simulink model "IP"  (R2023a)
settings: Solver=VariableStepAuto  StartTime=0.0  StopTime=25  FixedStep=0.1  RelTol=1e-3  AbsTol=1e-3  EnableMultiTasking=on
values from neighbouring files (symbols this model uses):
  A = [0 1 0 0 ... (first row only)    [IP_Parameters.m]
  B = [0;-1/(M*l);0;1/M]    [IP_Parameters.m]
  C = [1 0 1 0 ... (first row only)    [IP_Parameters.m]
  D = [0;0]    [IP_Parameters.m]
  g = 9.81    [IP_Parameters.m]
  kb = 0.031    [IP_Parameters.m]
  Kr = lqr(A,B,Q,R)    [IP_Parameters.m]
  kt = 0.031    [IP_Parameters.m]
  l = 0.36    [IP_Parameters.m]
  M = 2.4    [IP_Parameters.m]
  m = 0.23    [IP_Parameters.m]
  r = 0.006    [IP_Parameters.m]
  reg = lqg(sys,QXU,QWV,QI)    [IP_Parameters.m]
  Rm = 12.5    [IP_Parameters.m]
undefined symbols (not defined in the file or in its folder): b, c, Continuous, Discrete, I, K, KK, sysKF, Time, Vn, X, Y, Z
libraries: sm_lib x36, nesl_utility x20, simulink x14, vrlib x6, ctrlSharedLib x3, slpidlib x1
(part 1 of 2)
settings Model: Creator=M3tal  LastModifiedBy=M3tal
settings SolverCC: AutoScaleAbsTol=off  AlgebraicLoopSolver=TrustRegion  MaxZcPerStep=1
settings DataIOCC: LimitDataPoints=on  MaxDataPoints=10000
settings OptimizationCC: ReuseModelBlockBuffer=off  LifeSpan=inf
settings DebuggingCC: UnconnectedInputMsg=warning  UnconnectedOutputMsg=warning  UnconnectedLineMsg=warning  AllowSymbolicDim=off  SubsystemReferenceDiagnosticForUnitTest=warning  SFUnexpectedBacktrackingDiag=warning  SFNoUnconditionalDefaultTransitionDiag=warning  SFExecutionAtInitializationDiag=none  ArithmeticOperatorsInVariantConditions=warning
settings ModelReferenceCC: EnableRefExpFcnMdlSchedulingChecks=on
settings SFSimCC: SimUseLocalCustomCode=off  CustomCodeUndefinedFunction=UseInterfaceOnly
settings RTWCC: RTWUseLocalCustomCode=off  DLArmComputeVersion=19.05
settings CodeAppCC: StateflowObjectComments=on
settings GRTTargetCC: TargetLangStandard=C89/C90 (ANSI)
settings ConfigComp: CovMetricSettings=dw  CovSaveCumulativeToWorkspaceVar=on  CovSaveSingleToWorkspaceVar=on  CovExternalEMLEnable=off  CovSFcnEnable=off
settings SimscapeCC: SimscapeLogType=all  SimscapeLogSimulationStatistics=on  SimscapeLogDataHistory=10000
settings ExplorerConfigSet: InternalSimMechanicsExplorerSettings="<ExplorerConfiguration><canonicalview>default</canonicalview><AnimationSetting><BasePlaybackSpeed>1.0</BasePlaybackSpeed><PlaybackSpeedFactor>0.25</PlaybackSpeedFactor></AnimationSetting><TilePanel><TileInfo><Tiles Columns=\"1\" Count=\"1\" Rows=\"1\"><Column Weight=\"1\"/><Row Weight=\"1\"/><Tile Height=\"1\" Width=\"1\" X=\"0\" Y=\"0\"/></Tiles></TileInfo><SceneInfo><SceneViewer><BGColor><R>1</R><G>1</G><B>1</B></BGColor><Camera><DoPerspective>off</DoPerspective><Position><X>-0.0931380418765744289</X><Y>-1</Y><Z>0.280046106303800779</Z></Position><Center><X>-0.0931380418765744289</X><Y>-2.77555756156289135e-17</Y><Z>0.280046106303800779</Z></Center><Up><X>0</X><Y>-0</Y><Z>1</Z></Up><ViewLimDist>1</ViewLimDist><YLim>0.450745035862720633</YLim><XLim>0.829412650000000418</XLim></Camera></SceneViewer></SceneInfo></TilePanel><MechEditorPanel><Cameras/><GfxPanelCameraMap/><VideoCreator><PlaybackSpeedRatio>1.0</PlaybackSpeedRatio><FrameRate>30</FrameRate><VideoFormat>Motion JPEG AVI</VideoFormat><FrameSize>auto</FrameSize></VideoCreator></MechEditorPanel></ExplorerConfiguration>"

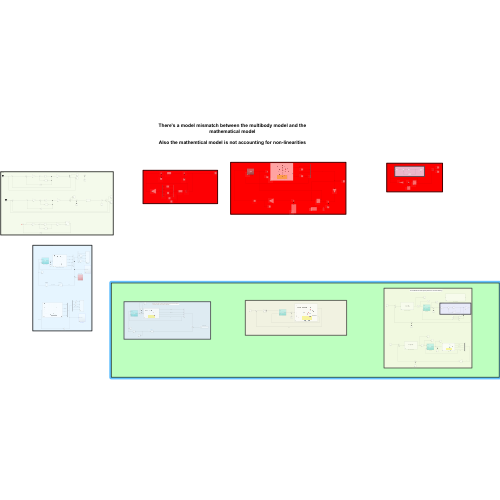
[thumbnail: Simulink's stored preview of the top-level diagram]
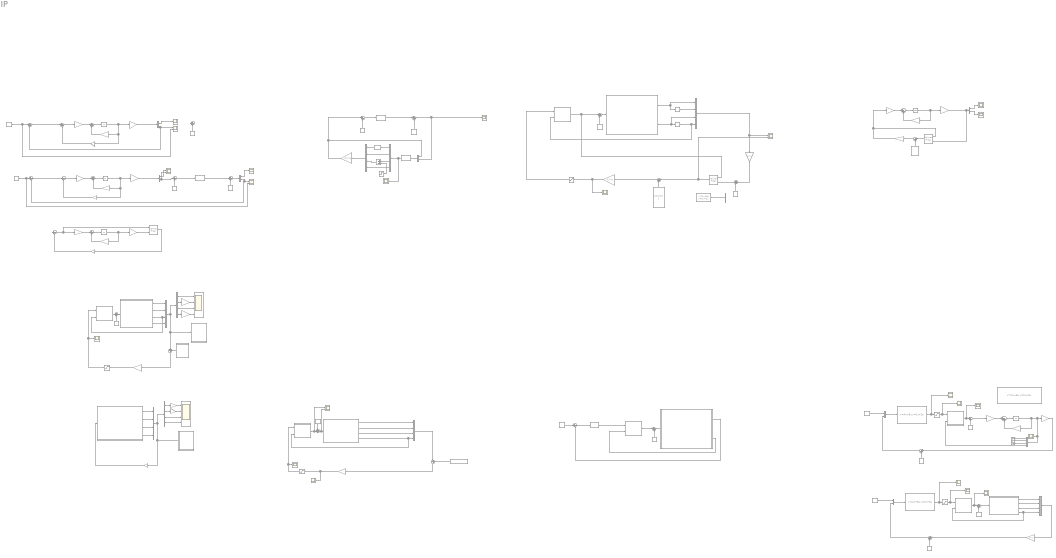
== system IP ==
  note: There's a model mismatch between the multibody model and the mathematical model
      |
      | Also the mathemtical model is not accounting for non-linearities
  note: the model with the state space plant is the one that's working
  note: LQG
  note: Obsolete
  note: nonlinear models in simulink blocks with LQR that i stole
  note: LQG but the G and H matrix are needed
  note: LQG using LQR and KF
  note: LQG Acceptable Results following steve brunton lqg example
  note: PID
  note: When the noise power is incresed the pendulum swerve largely and it loses it's linearzed charecterisitics and the controller doesn't act appropiately
  note: LQR
  note: Plant
  note: Plant
  3D Animation : Subsystem  Commented=on
  3D Animation1 : Subsystem  Commented=on
  Actautor : Subsystem  Commented=on
  Actautor1 : Subsystem  Commented=on
  Actautor2 : Subsystem  Commented=on
  Actautor3 : Subsystem  Commented=on
  Add : Sum  Commented=on  Inputs=+-
  Band-Limited White Noise : simulink/Sources/Band-Limited White Noise  Commented=on  Cov=[1]  Ts=0.1  seed=[23341]
  Band-Limited White Noise{1..2,4,6,11,16..17} (7 alike) : simulink/Sources/Band-Limited White Noise  Commented=on  Cov=[0.1]  Ts=0.1  seed=[23341]
  Band-Limited White Noise{5,8..10} (4 alike) : simulink/Sources/Band-Limited White Noise  Commented=on  Cov=0.1  Ts=0.1  seed=[23341]
  Band-Limited White Noise24 : simulink/Sources/Band-Limited White Noise  Commented=on  Cov=[2]  Ts=0.1  seed=[23341]
  Band-Limited White Noise7 : simulink/Sources/Band-Limited White Noise  Commented=on  Cov=[0.5]  Ts=0.1  seed=[23341]
  Bias1 : Bias  Commented=on  SaturateOnIntegerOverflow=off
  Constant : Constant  Commented=on  Value=[0 0]
  Constant1 : Constant  Commented=on  Value=0
  Constant2 : Constant  Commented=on  Value=[ 0 0 0 0 ]
  Constant3 : Constant  Commented=on  Value=[0 0]
  Demux{,1,3,8} (4 alike) : Demux  Commented=on  Outputs=2
  Demux{4,12..14} (4 alike) : Demux  Commented=on
  Derivative8 : Derivative  Commented=on
  Derivative9 : Derivative  Commented=on
  Desire_state : Subsystem  Commented=on
  Desired state : Constant  Commented=on  Value=[ 0 0 0 0]
  Gain : Gain  Commented=on  Gain=C  Multiplication=Matrix(K*u) (u vector)
  Gain{1,4,9,16,21} (5 alike) : Gain  Commented=on  Gain=A  Multiplication=Matrix(K*u)
  Gain{2,5,10,17,23} (5 alike) : Gain  Commented=on  Gain=C  Multiplication=Matrix(K*u)
  Gain{3,6,11,18,24} (5 alike) : Gain  Commented=on  Gain=B  Multiplication=Matrix(K*u)
  Gain12 : Gain  Commented=on  Gain=K  Multiplication=Matrix(K*u)
  Gain15 : Gain  Commented=on  Gain=Kr  Multiplication=Matrix(K*u) (u vector)
  Gain19 : Gain  Commented=on  Gain=Kr  Multiplication=Matrix(K*u)
  Gain22 : Gain  Commented=on  Gain=-Kr  Multiplication=Matrix(K*u)
  Gain27 : Gain  Commented=on  Gain=Kr  Multiplication=Matrix(K*u) (u vector)
  Gain28 : Gain  Commented=on  Gain=C  Multiplication=Matrix(K*u) (u vector)
  Gain29 : Gain  Commented=on  Gain=KK  Multiplication=Matrix(K*u)
  Gain7 : Gain  Commented=on  Gain=K  Multiplication=Matrix(K*u)
  Gain8 : Gain  Commented=on  Gain=K  Multiplication=Matrix(K*u)
  INPUT : Scope  Commented=on
  IP model using ss : StateSpace  Commented=on  A=A  B=B  C=C  D=D  InitialCondition=0
  Integrator{1..4,6} (5 alike) : Integrator  Commented=on
  Inverted Pendulum System : Subsystem  Commented=on
      mask Display: image('ip_model.png');
  Inverted Pendulum System1 : Subsystem  Commented=on
      mask Display: image('ip_model.png');
  KF using matlab : StateSpace  Commented=on  A=sysKF.A  B=sysKF.B  C=sysKF.C  D=sysKF.D  InitialCondition=0
  KF1 : StateSpace  Commented=on  A=sysKF.A  B=sysKF.B  C=sysKF.C  D=sysKF.D  InitialCondition=0
  Kalman Filter : ctrlSharedLib/Kalman Filter  Commented=on  TimeDomain=Discrete-Time  UseCurrentEstimator=on  ModelSource=LTI State-Space Variable  ModelSourceVariable=ss(0.95,1,1,0,1)  A=0.95  B=1  C=1  D=0  NumberOfStates=1  NumberOfInputs=1  NumberOfOutputs=1  InitialEstimateSource=Dialog  X0=0  P0=10  UseK=off  UseGH=off  NumberOfProcessNoiseInputs=1  G=1  TimeInvariantG=on  H=0  TimeInvariantH=on  Q=0.05  TimeInvariantQ=on  R=1  TimeInvariantR=on  N=0  TimeInvariantN=on  AddInputPort=on  AddEnablePort=off  OutputEstimatedY=off  OutputP=off  Ts=-1
  Kalman Filter1 : ctrlSharedLib/Kalman Filter  Commented=on  TimeDomain=Continuous-Time  UseCurrentEstimator=on  ModelSource=Individual A, B, C, D matrices  ModelSourceVariable=ss(0.95,1,1,0,1)  A=A  B=B  C=C  D=D  NumberOfStates=1  NumberOfInputs=1  NumberOfOutputs=1  InitialEstimateSource=Dialog  X0=0  P0=10  UseK=off  UseGH=off  NumberOfProcessNoiseInputs=1  G=1  TimeInvariantG=on  H=0  TimeInvariantH=on  Q=Vd  TimeInvariantQ=on  R=Vn  TimeInvariantR=on  N=0  TimeInvariantN=on  AddInputPort=on  AddEnablePort=off  OutputEstimatedY=off  OutputP=off  Ts=-1
  Kalman Filter3 : ctrlSharedLib/Kalman Filter  Commented=on  TimeDomain=Continuous-Time  UseCurrentEstimator=on  ModelSource=Individual A, B, C, D matrices  ModelSourceVariable=ss(0.95,1,1,0,1)  A=A  B=B  C=C  D=D  NumberOfStates=1  NumberOfInputs=1  NumberOfOutputs=1  InitialEstimateSource=Dialog  X0=0  P0=10  UseK=off  UseGH=off  NumberOfProcessNoiseInputs=1  G=1  TimeInvariantG=on  H=0  TimeInvariantH=on  Q=0.07  TimeInvariantQ=on  R=1  TimeInvariantR=on  N=0  TimeInvariantN=on  AddInputPort=on  AddEnablePort=off  OutputEstimatedY=off  OutputP=off  Ts=-1
  LQG servo controller : StateSpace  Commented=on  A=reg.A  B=reg.B  C=reg.C  D=reg.D  InitialCondition=0
  LQG servo controller1 : StateSpace  Commented=on  A=reg.A  B=reg.B  C=reg.C  D=reg.D  InitialCondition=0
  LQR_Gain : Gain  Commented=on  Gain=KK  Multiplication=Matrix(K*u)
  Mux{,1,12..13,15,17} (6 alike) : Mux  Commented=on
  Mux{2,5,10..11} (4 alike) : Mux  Commented=on  Inputs=2
  OUTPUT : Scope  Commented=on  NumInputPorts=4
  OUTPUT1 : Scope  Commented=on  NumInputPorts=4
  PID Controller : slpidlib/PID Controller  Commented=on  Controller=PID  Form=Parallel  TimeDomain=Continuous-time  UseExternalTs=off  SampleTime=-1  IntegratorMethod=Forward Euler  FilterMethod=Forward Euler  ControllerParametersSource=internal  P=-3207.65217868692  I=-1870.9153966155  UseKiTs=off  D=-19.0235650193151  N=66.8915557293185  UseFilter=on  TunerSelectOption=Transfer Function Based (PID Tuner App)  InitialConditionSource=internal  InitialConditionForIntegrator=0  InitialConditionForFilter=0  DifferentiatorICPrevScaledInput=0  ExternalReset=none  TrackingMode=off  Kt=1  LimitOutput=on  SatLimitsSource=internal  UpperSaturationLimit=24  LowerSaturationLimit=-24  LinearizeAsGain=on  AntiWindupMode=clamping  Kb=1  LimitIntegrator=off  UpperIntegratorSaturationLimit=24  LowerIntegratorSaturationLimit=-24  POutMin=[]  POutMax=[]  IOutMin=[]  IOutMax=[]  DOutMin=[]  DOutMax=[]  NOutMin=[]  NOutMax=[]  SumOutMin=[]  SumOutMax=[]  SaturationOutMin=[]  SaturationOutMax=[]  PParamMin=[]  PParamMax=[]  IParamMin=[]  IParamMax=[]  DParamMin=[]  DParamMax=[]  NParamMin=[]  NParamMax=[]  KbParamMin=[]  KbParamMax=[]  KtParamMin=[]  KtParamMax=[]  KbOutMin=[]  KbOutMax=[]  KtOutMin=[]  KtOutMax=[]  IntegratorOutMin=[]  IntegratorOutMax=[]  FilterOutMin=[]  FilterOutMax=[]  SumI1OutMin=[]  SumI1OutMax=[]  SumI2OutMin=[]  SumI2OutMax=[]  SumI3OutMin=[]  SumI3OutMax=[]  SumI4OutMin=[]  SumI4OutMax=[]  SumDOutMin=[]  SumDOutMax=[]  DifferentiatorOutMin=[]  DifferentiatorOutMax=[]  FilterDiffOutCoefMin=[]  FilterDiffOutCoefMax=[]  ReciprocalOutMin=[]  ReciprocalOutMax=[]  SumDenOutMin=[]  SumDenOutMax=[]  SumNumOutMin=[]  SumNumOutMax=[]  DivideOutMin=[]  DivideOutMax=[]  UdiffTsProdOutMin=[]  UdiffTsProdOutMax=[]  NTsProdOutMin=[]  NTsProdOutMax=[]  UintegralTsProdOutMin=[]  UintegralTsProdOutMax=[]  UngainTsProdOutMin=[]  UngainTsProdOutMax=[]  ClampingZeroOutDataTypeStr=Inherit: Inherit via back propagation  ClampingZeroOutMin=[]  ClampingZeroOutMax=[]  FilterDenConstantOutDataTypeStr=Inherit: Inherit via back propagation  FilterDenConstantOutMin=[]  FilterDenConstantOutMax=[]  PCopyOutDataTypeStr=Inherit: Inherit via back propagation  PCopyOutMin=[]  PCopyOutMax=[]  NCopyOutDataTypeStr=Inherit: Inherit via back propagation  NCopyOutMin=[]  NCopyOutMax=[]  IntegratorContinuousStateAttributes=''  IntegratorStateMustResolveToSignalObject=off  IntegratorRTWStateStorageClass=Auto  FilterContinuousStateAttributes=''  FilterStateMustResolveToSignalObject=off  FilterRTWStateStorageClass=Auto  ParallelPVariant=InternalParameters  IdealPVariant=Disabled  IVariant=InternalParameters  DVariant=InternalParameters  IntegratorVariant=Continuous  SatVariant=Enabled  AWVariant=ContClampingParallel  PCopyVariant=Disabled  TRVariant=Disabled  FdbkBlocksVariant=Forward  IdealPFdbkVariant=Disabled  SatFdbkVariant=Disabled  DerivativeFilterVariant=ContFilter  NVariant=InternalParameters  NCopyVariant=Disabled  FilterICVariant=InternalICsFilter  IntegratorICVariant=InternalICs  ExternalResetVariant=Disabled  TRSumVariant=Passthrough  SumFdbkVariant=Disabled  SumVariant=Sum_PID  TsampFilterVariant=InternalTs  TsampNgainVariant=Passthrough  TsampIntegralVariant=Disabled_SignalSpec  ExternalSaturationOutDataTypeStr=Inherit: Same as second input
  Plant : Subsystem  Commented=on
      mask Display: image('Annotation 2024-07-04 030345.png'); % Use "Edit Image" on toolstrip to change.
  Plant1 : Subsystem  Commented=on
      mask Display: image('Annotation 2024-07-04 030345.png'); % Use "Edit Image" on toolstrip to change.
  Plant2 : Subsystem  Commented=on
      mask Display: image('Annotation 2024-07-04 030345.png'); % Use "Edit Image" on toolstrip to change.
  Plant9 : Subsystem  Commented=on
      mask Display: image('Annotation 2024-07-04 030345.png'); % Use "Edit Image" on toolstrip to change.
  Plant_in_SSblock : StateSpace  Commented=on  A=A  B=B  C=C  D=D  InitialCondition=0
  R2D : Gain  Commented=on  Gain=180/pi
  R2D1 : Gain  Commented=on  Gain=180/pi
  REf Vs x : Scope  Commented=on  NumInputPorts=2
  Radian_to_Degre : Gain  Commented=on  Gain=180/pi
  Radian_to_Degree : Gain  Commented=on  Gain=180/pi
  Saturation{,1..3} (4 alike) : Saturate  Commented=on  UpperLimit=24  LowerLimit=-24
  Scope{,1,9,18} (4 alike) : Scope  Commented=on  NumInputPorts=2
  Scope{3..8,10..12,14..17,19} (14 alike) : Scope  Commented=on
  Signal Generator : SignalGenerator  Commented=on  WaveForm=square  Units=rad/sec
  Signal Generator1 : SignalGenerator  Commented=on  WaveForm=square  Units=rad/sec
  State-Space : StateSpace  Commented=on  A=A  B=B  C=C  D=D  InitialCondition=0
  Step : Step  Commented=on  Time=10  After=20  SampleTime=0
  Sum{,2..4,8..9,13,15..16,20..22,24..25,33..34,43,46} (18 alike) : Sum  Commented=on  Inputs=|++
  Sum{1,5..7,11..12} (6 alike) : Sum  Commented=on  Inputs=|+-
  Sum{14,17,19,45} (4 alike) : Sum  Commented=on  Inputs=|-+
  Sum18 : Sum  Commented=on  Inputs=++|
  Terminator : Terminator  Commented=on
  Terminator1 : Terminator  Commented=on
  Terminator2 : Terminator  Commented=on
  Volatge_to_Force : Subsystem  Commented=on
  Volatge_to_Force1 : Subsystem  Commented=on
  Voltage Saturation : Saturate  Commented=on  UpperLimit=24  LowerLimit=-24
  Zero : Constant  Commented=on  Value=[ 0 0 0 0]  OutDataTypeStr=Inherit: Inherit via back propagation
  theta : Scope  Commented=on
  theta2 : Scope  Commented=on
  wires:
  Sum1/1 -> PID Controller/1
  Constant1/1 -> Sum1/1
  Signal Generator/1 -> Sum5/1, REf Vs x/2
  State-Space/1 -> Sum4/1
  Band-Limited White Noise1/1 -> Sum4/2
  Sum4/1 -> Demux/1
  Demux/1 -> theta/1
  Demux/2 -> Sum5/2, REf Vs x/1
  ? -> Sum6/1
  Gain6/1 -> Sum3/1
  Gain4/1 -> Sum3/2
  Integrator1/1 -> Gain4/1, Gain5/1  "X"
  Sum3/1 -> Integrator1/1  "X-dot"
  Sum6/1 -> Kalman Filter/1, Gain6/1  "U"
  Gain7/1 -> Sum6/2
  Sum/1 -> State-Space/1
  Band-Limited White Noise2/1 -> Sum/2
  Gain2/1 -> Demux1/1
  Gain8/1 -> Sum7/2
  Sum7/1 -> Gain3/1
  Sum2/1 -> Integrator2/1
  Integrator2/1 -> Gain2/1, Gain8/1, Gain1/1
  Gain1/1 -> Sum2/2
  Gain3/1 -> Sum2/1
  Sum5/1 -> Sum7/1
  Demux1/2 -> Sum/1, Scope/2
  Demux1/1 -> Scope/1
  Sum11/1 -> Sum12/1
  Gain11/1 -> Sum9/1
  Gain9/1 -> Sum9/2
  Integrator3/1 -> Gain9/1, Gain12/1, Gain10/1
  Sum9/1 -> Integrator3/1
  Sum12/1 -> Gain11/1
  Gain12/1 -> Sum12/2
  Gain10/1 -> Demux3/1
  Band-Limited White Noise4/1 -> Sum8/2
  Signal Generator1/1 -> Scope1/2, Sum11/1
  Demux3/1 -> theta2/1
  Demux3/2 -> Sum11/2, Scope1/1
  Plant/1(Theta) -> Sum1/2  "Theta"
  Gain5/1 -> Kalman Filter/2  "Y"
  Kalman Filter/1 -> Gain7/1
  Plant2/1(Theta) -> Mux1/1  "Theta"
  Sum18/1 -> Scope9/2, Plant2/1(Force)
  Integrator4/1 -> Gain17/1, Gain16/1
  Gain18/1 -> Sum24/1
  Sum24/1 -> Integrator4/1
  Kalman Filter3/1 -> Sum14/1
  Demux8/1 -> Scope6/1
  Gain19/1 -> Gain18/1, Kalman Filter3/1
  LQG servo controller/1 -> Scope3/1, Saturation2/1
  Gain17/1 -> Kalman Filter3/2, Demux8/1  "y"
  Demux8/2 -> Scope8/1
  Demux12/3 -> Add/1  "x"
  Mux11/1 -> KF1/1
  Mux12/1 -> Gain22/1  "X_hat"
  Gain22/1 -> Sum33/1, Mux11/1  "u"
  Demux12/4 -> Mux12/4  "x_dot"
  Demux12/1 -> Bias1/1  "Theta"
  Bias1/1 -> Mux12/1
  Demux12/2 -> Mux12/2  "Theta_dot"
  KF1/1 -> Scope15/1, Demux12/1  "X_hat"
  Step/1 -> Add/2
  Add/1 -> Mux12/3
  Sum33/1 -> IP model using ss/1
  Band-Limited White Noise16/1 -> Sum33/2
  Band-Limited White Noise17/1 -> Sum34/2
  Sum34/1 -> Mux11/2, Scope12/1  "y"
  IP model using ss/1 -> Sum34/1  "y"
  Volatge_to_Force1/1(Force (N)) -> Kalman Filter1/1, Sum20/1  "u"
  Plant9/1(Theta) -> Mux17/1, Derivative8/1  "Theta"
  Mux17/1 -> Gain28/1, Scope18/1  "X"
  Derivative8/1 -> Mux17/2  "Theta_dot"
  Plant9/2(x) -> Mux17/3, Derivative9/1  "x"
  Derivative9/1 -> Volatge_to_Force1/2(X_dot), Mux17/4  "x_dot"
  Gain28/1 -> Sum43/1  "y"
  Mux10/1 -> KF using matlab/1
  Demux13/1 -> R2D/1
  Demux13/4 -> OUTPUT/4
  Demux13/3 -> OUTPUT/3
  Gain29/1 -> Inverted Pendulum System/1(Force)  "Input_Force"
  Mux13/1 -> Demux13/1, Gain29/1, 3D Animation/1(3D Animation)
  Inverted Pendulum System/2(theta_dot) -> Mux13/2  "theta_dot"
  Demux13/2 -> Radian_to_Degre/1
  Inverted Pendulum System/1(theta) -> Mux13/1  "theta"
  Inverted Pendulum System/3(x) -> Mux13/3  "X"
  Inverted Pendulum System/4(x_dot) -> Mux13/4  "X_dot"
  R2D/1 -> OUTPUT/1
  Radian_to_Degre/1 -> OUTPUT/2
  Volatge_to_Force/1(Force (N)) -> Sum46/1
  Band-Limited White Noise24/1 -> Sum46/2
  Sum46/1 -> Inverted Pendulum System1/1(Force)
  Radian_to_Degree/1 -> OUTPUT1/4
  Demux14/4 -> Radian_to_Degree/1
  Demux14/3 -> OUTPUT1/3
  Demux14/2 -> R2D1/1
  Demux14/1 -> OUTPUT1/1
  Inverted Pendulum System1/2(theta) -> Mux15/2  "theta"
  Inverted Pendulum System1/1(x) -> Mux15/1  "X"
  LQR_Gain/1 -> Voltage Saturation/1  "Motor_voltage"
  R2D1/1 -> OUTPUT1/2
  Inverted Pendulum System1/3(x_dot) -> Volatge_to_Force/2(X_dot), Mux15/3  "X_dot"
  Desire_state/1(X) -> Sum45/2
  Inverted Pendulum System1/4(theta_dot) -> Mux15/4  "theta_dot"
  Voltage Saturation/1 -> INPUT/1, Volatge_to_Force/1(Voltage)
  Mux1/1 -> Sum17/1
  Desired state/1 -> Sum17/2
  Band-Limited White Noise/1 -> Sum13/2
  Sum13/1 -> Plant/1(Force)
  Plant/2(Output) -> Actautor/2(X_dot)
  Actautor/1(Force (N)) -> Sum13/1
  PID Controller/1 -> Actautor/1(Voltage)
  Sum17/1 -> Gain15/1
  Gain15/1 -> Scope7/1, Saturation/1  "LQR gain"
  Actautor1/1(Force (N)) -> Scope9/1, Sum18/2
  Saturation/1 -> Actautor1/1(Voltage), Scope4/1
  Sum45/1 -> LQR_Gain/1  "-(X - X_d)"
  Mux15/1 -> Demux14/1, Sum45/1, 3D Animation1/1(3D Animation)
  Constant2/1 -> Sum19/2
  Sum19/1 -> Gain27/1
  Kalman Filter1/1 -> Scope18/2, Sum19/1
  Gain27/1 -> Saturation1/1, Scope17/1
  Sum20/1 -> Plant9/1(Force)
  Band-Limited White Noise8/1 -> Sum20/2
  Band-Limited White Noise9/1 -> Sum43/2
  Sum43/1 -> Kalman Filter1/2
  Saturation1/1 -> Volatge_to_Force1/1(Voltage)
  Zero/1 -> Sum14/2
  Sum14/1 -> Gain19/1
  Gain16/1 -> Sum24/2
  Band-Limited White Noise5/1 -> Sum15/2
  Actautor2/1(Force (N)) -> Scope10/1, Sum15/1
  Sum15/1 -> Plant1/1(Force)
  Saturation2/1 -> Scope5/1, Actautor2/1(Voltage)
  Mux/1 -> Gain/1  "x"
  Gain/1 -> Sum21/1  "y"
  Mux2/1 -> LQG servo controller/1
  Constant/1 -> Mux2/1
  Sum21/1 -> Mux2/2
  Band-Limited White Noise6/1 -> Sum21/2
  Saturation3/1 -> Scope16/1, Actautor3/1(Voltage)
  Actautor3/1(Force (N)) -> Scope11/1, Sum16/1
  Band-Limited White Noise10/1 -> Sum16/2
  Mux5/1 -> LQG servo controller1/1
  Sum16/1 -> Gain24/1
  Constant3/1 -> Mux5/1
  Sum22/1 -> Mux5/2
  LQG servo controller1/1 -> Scope14/1, Saturation3/1
  Band-Limited White Noise11/1 -> Sum22/2
  Gain21/1 -> Sum25/2
  Integrator6/1 -> Demux4/1, Scope19/1, Gain23/1, Gain21/1  "X"
  Sum25/1 -> Integrator6/1
  Gain24/1 -> Sum25/1
  Gain23/1 -> Sum22/1  "y"
  Demux4/1 -> Terminator2/1
  Demux4/2 -> Terminator1/1
  Demux4/4 -> Actautor3/2(X_dot)
  Demux4/3 -> Terminator/1
  Plant2/2(Theta_dot) -> Mux1/2  "Theta_dot"
  Plant2/3(x) -> Mux1/3  "x"
  Plant2/4(x_dot) -> Actautor1/2(X_dot), Mux1/4  "x_dot"
  Band-Limited White Noise7/1 -> Sum18/1
  Plant1/3(x) -> Mux/3  "x"
  Plant1/1(Theta) -> Mux/1  "Theta"
  Plant1/2(Theta_dot) -> Mux/2  "Theta_dot"
  Plant1/4(x_dot) -> Actautor2/2(X_dot), Mux/4  "x_dot"

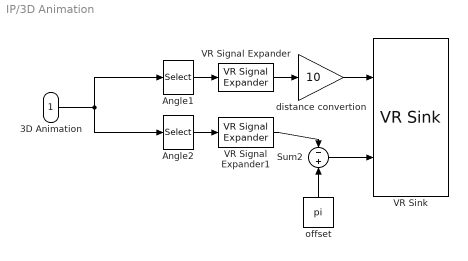
== system IP/3D Animation ==
  3D Animation : Inport
  Angle1 : Selector  InputPortWidth=4  IndexOptions=Index vector (dialog)  Indices=[1]  OutputSizes=1
  Angle2 : Selector  InputPortWidth=4  IndexOptions=Index vector (dialog)  Indices=[2]  OutputSizes=1
  Sum2 : Sum  Inputs=-|+
  VR Signal Expander : vrlib/VR Signal Expander  outwidth=3  outidx=[1]
  VR Signal Expander1 : vrlib/VR Signal Expander  outwidth=4  outidx=[4]
  VR Sink : vrlib/VR Sink  InstantiateOnLoad=on  SampleTime=0.02  ViewEnable=on  RemoteChange=off  RemoteView=off  FieldsWritten=cart.translation.3.1.1.double#joint.rotation.4.1.1.double  WorldFileName=Inverted_pendulum12.wrl  AutoView=off  VideoDimensions=[]  AllowVariableSize=off  FigureProperties=[]
  distance convertion : Gain  Gain=10
  offset : Constant  Value=pi
  wires:
  VR Signal Expander/1 -> distance convertion/1
  3D Animation/1 -> Angle2/1, Angle1/1
  Angle1/1 -> VR Signal Expander/1
  Angle2/1 -> VR Signal Expander1/1
  offset/1 -> Sum2/2
  Sum2/1 -> VR Sink/2
  VR Signal Expander1/1 -> Sum2/1
  distance convertion/1 -> VR Sink/1

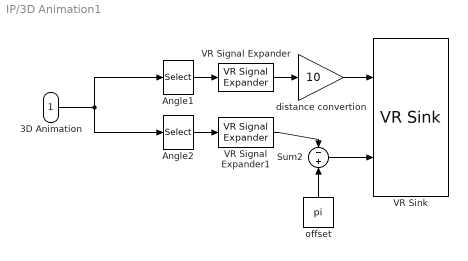
== system IP/3D Animation1 ==
  3D Animation : Inport
  Angle1 : Selector  InputPortWidth=4  IndexOptions=Index vector (dialog)  Indices=[1]  OutputSizes=1
  Angle2 : Selector  InputPortWidth=4  IndexOptions=Index vector (dialog)  Indices=[2]  OutputSizes=1
  Sum2 : Sum  Inputs=-|+
  VR Signal Expander : vrlib/VR Signal Expander  outwidth=3  outidx=[1]
  VR Signal Expander1 : vrlib/VR Signal Expander  outwidth=4  outidx=[4]
  VR Sink : vrlib/VR Sink  InstantiateOnLoad=on  SampleTime=0.02  ViewEnable=on  RemoteChange=off  RemoteView=off  FieldsWritten=cart.translation.3.1.1.double#joint.rotation.4.1.1.double  WorldFileName=Inverted_pendulum12.wrl  AutoView=off  VideoDimensions=[]  AllowVariableSize=off  FigureProperties=[]
  distance convertion : Gain  Gain=10
  offset : Constant  Value=pi
  wires:
  VR Signal Expander/1 -> distance convertion/1
  3D Animation/1 -> Angle2/1, Angle1/1
  Angle1/1 -> VR Signal Expander/1
  Angle2/1 -> VR Signal Expander1/1
  offset/1 -> Sum2/2
  Sum2/1 -> VR Sink/2
  VR Signal Expander1/1 -> Sum2/1
  distance convertion/1 -> VR Sink/1

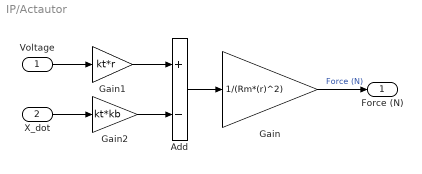
== system IP/Actautor ==
  Voltage : Inport
  X_dot : Inport  Port=2
  Add : Sum  Inputs=+-
  Gain : Gain  Gain=1/(Rm*(r)^2)
  Gain1 : Gain  Gain=kt*r
  Gain2 : Gain  Gain=kt*kb
  Force (N) : Outport  VectorParamsAs1DForOutWhenUnconnected=off
  wires:
  Gain1/1 -> Add/1
  Gain2/1 -> Add/2
  Voltage/1 -> Gain1/1
  Gain/1 -> Force (N)/1  "Force (N)"
  X_dot/1 -> Gain2/1
  Add/1 -> Gain/1

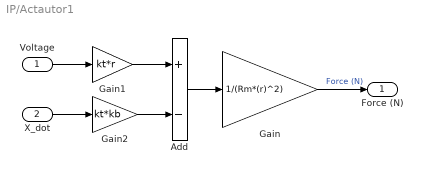
== system IP/Actautor1 ==
  Voltage : Inport
  X_dot : Inport  Port=2
  Add : Sum  Inputs=+-
  Gain : Gain  Gain=1/(Rm*(r)^2)
  Gain1 : Gain  Gain=kt*r
  Gain2 : Gain  Gain=kt*kb
  Force (N) : Outport  VectorParamsAs1DForOutWhenUnconnected=off
  wires:
  Add/1 -> Gain/1
  X_dot/1 -> Gain2/1
  Gain/1 -> Force (N)/1  "Force (N)"
  Voltage/1 -> Gain1/1
  Gain2/1 -> Add/2
  Gain1/1 -> Add/1

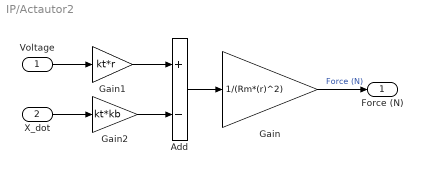
== system IP/Actautor2 ==
  Voltage : Inport
  X_dot : Inport  Port=2
  Add : Sum  Inputs=+-
  Gain : Gain  Gain=1/(Rm*(r)^2)
  Gain1 : Gain  Gain=kt*r
  Gain2 : Gain  Gain=kt*kb
  Force (N) : Outport  VectorParamsAs1DForOutWhenUnconnected=off
  wires:
  Add/1 -> Gain/1
  X_dot/1 -> Gain2/1
  Gain/1 -> Force (N)/1  "Force (N)"
  Voltage/1 -> Gain1/1
  Gain2/1 -> Add/2
  Gain1/1 -> Add/1

== system IP/Actautor3 ==
  Voltage : Inport
  X_dot : Inport  Port=2
  Add : Sum  Inputs=+-
  Gain : Gain  Gain=1/(Rm*(r)^2)
  Gain1 : Gain  Gain=kt*r
  Gain2 : Gain  Gain=kt*kb
  Force (N) : Outport  VectorParamsAs1DForOutWhenUnconnected=off
  wires:
  Add/1 -> Gain/1
  X_dot/1 -> Gain2/1
  Gain/1 -> Force (N)/1  "Force (N)"
  Voltage/1 -> Gain1/1
  Gain2/1 -> Add/2
  Gain1/1 -> Add/1

== system IP/Desire_state ==
  Angle_D(rad) : Constant  Value=pi
  Mux1 : Mux
  Position_dot_D(m/sec) : Constant  Value=0
  Position_dot_D(m/sec)1 : Constant  Value=0
  angle_dot_D(rad/sec) : Constant  Value=0
  X : Outport  VectorParamsAs1DForOutWhenUnconnected=off
  wires:
  Mux1/1 -> X/1
  Position_dot_D(m/sec)/1 -> Mux1/3
  angle_dot_D(rad/sec)/1 -> Mux1/4
  Angle_D(rad)/1 -> Mux1/2
  Position_dot_D(m/sec)1/1 -> Mux1/1

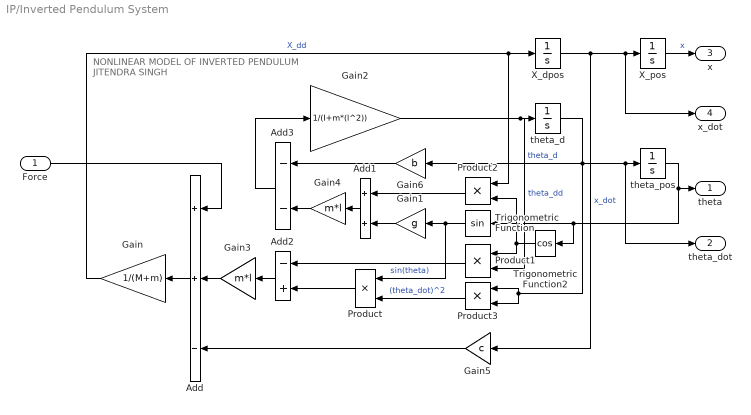
== system IP/Inverted Pendulum System ==
  note: NONLINEAR MODEL OF
      | INVERTED PENDULUM
      | JITENDRA SINGH
  Force : Inport
  Add : Sum  Inputs=++-
  Add1 : Sum
  Add2 : Sum  Inputs=-+
  Add3 : Sum  Inputs=--
  Gain : Gain  Gain=1/(M+m)
  Gain1 : Gain  Gain=g
  Gain2 : Gain  Gain=1/(I+m*(l^2))
  Gain3 : Gain  Gain=m*l
  Gain4 : Gain  Gain=m*l
  Gain5 : Gain  Gain=c
  Gain6 : Gain  Gain=b
  Product{,1..3} (4 alike) : Product
  Trigonometric Function : Trigonometry
  Trigonometric Function2 : Trigonometry  Operator=cos
  X_dpos : Integrator
  X_pos : Integrator
  theta_d : Integrator
  theta_pos : Integrator  InitialCondition=45*(pi/180)
  theta : Outport  VectorParamsAs1DForOutWhenUnconnected=off
  theta_dot : Outport  Port=2  VectorParamsAs1DForOutWhenUnconnected=off
  x : Outport  Port=3  VectorParamsAs1DForOutWhenUnconnected=off
  x_dot : Outport  Port=4  VectorParamsAs1DForOutWhenUnconnected=off
  wires:
  Gain5/1 -> Add/3
  Add2/1 -> Gain3/1
  Add3/1 -> Gain2/1
  Trigonometric Function2/1 -> Product2/2, Product1/1
  Trigonometric Function/1 -> Product/1, Gain1/1  "sin(theta)"
  Gain3/1 -> Add/2
  theta_d/1 -> Product3/2, Product3/1, Gain6/1, theta_dot/1, theta_pos/1  "theta_d"
  Product2/1 -> Add1/1
  Product/1 -> Add2/2
  Gain4/1 -> Add3/2
  Product3/1 -> Product/2  "(theta_dot)^2"
  X_pos/1 -> x/1  "x"
  Product1/1 -> Add2/1
  Gain/1 -> X_dpos/1, Product2/1  "X_dd"
  Add/1 -> Gain/1
  Gain2/1 -> Product1/2, theta_d/1  "theta_dd"
  Gain6/1 -> Add3/1
  theta_pos/1 -> Trigonometric Function2/1, Trigonometric Function/1, theta/1
  Force/1 -> Add/1
  Gain1/1 -> Add1/2
  X_dpos/1 -> x_dot/1, X_pos/1, Gain5/1  "x_dot"
  Add1/1 -> Gain4/1

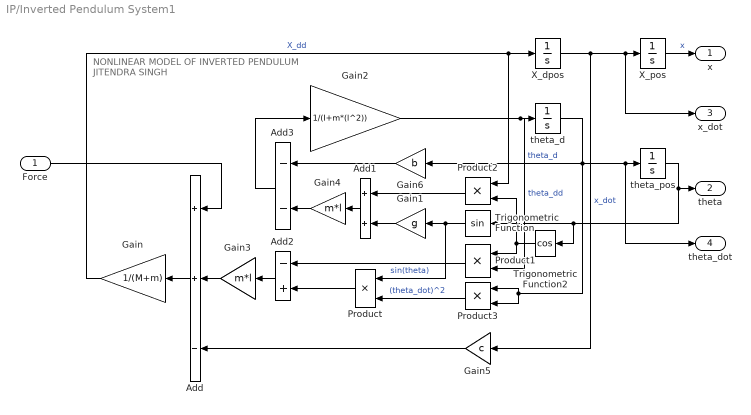
== system IP/Inverted Pendulum System1 ==
  note: NONLINEAR MODEL OF
      | INVERTED PENDULUM
      | JITENDRA SINGH
  Force : Inport
  Add : Sum  Inputs=++-
  Add1 : Sum
  Add2 : Sum  Inputs=-+
  Add3 : Sum  Inputs=--
  Gain : Gain  Gain=1/(M+m)
  Gain1 : Gain  Gain=g
  Gain2 : Gain  Gain=1/(I+m*(l^2))
  Gain3 : Gain  Gain=m*l
  Gain4 : Gain  Gain=m*l
  Gain5 : Gain  Gain=c
  Gain6 : Gain  Gain=b
  Product{,1..3} (4 alike) : Product
  Trigonometric Function : Trigonometry
  Trigonometric Function2 : Trigonometry  Operator=cos
  X_dpos : Integrator
  X_pos : Integrator  InitialCondition=0.2
  theta_d : Integrator
  theta_pos : Integrator  InitialCondition=160*(pi/180)
  x : Outport  VectorParamsAs1DForOutWhenUnconnected=off
  theta : Outport  Port=2  VectorParamsAs1DForOutWhenUnconnected=off
  x_dot : Outport  Port=3  VectorParamsAs1DForOutWhenUnconnected=off
  theta_dot : Outport  Port=4  VectorParamsAs1DForOutWhenUnconnected=off
  wires:
  Gain5/1 -> Add/3
  Add2/1 -> Gain3/1
  Add3/1 -> Gain2/1
  Trigonometric Function2/1 -> Product2/2, Product1/1
  Trigonometric Function/1 -> Product/1, Gain1/1  "sin(theta)"
  Gain3/1 -> Add/2
  theta_d/1 -> Product3/2, Product3/1, Gain6/1, theta_dot/1, theta_pos/1  "theta_d"
  Product2/1 -> Add1/1
  Product/1 -> Add2/2
  Gain4/1 -> Add3/2
  Product3/1 -> Product/2  "(theta_dot)^2"
  X_pos/1 -> x/1  "x"
  Product1/1 -> Add2/1
  Gain/1 -> X_dpos/1, Product2/1  "X_dd"
  Add/1 -> Gain/1
  Gain2/1 -> Product1/2, theta_d/1  "theta_dd"
  Gain6/1 -> Add3/1
  theta_pos/1 -> Trigonometric Function2/1, Trigonometric Function/1, theta/1
  Force/1 -> Add/1
  Gain1/1 -> Add1/2
  X_dpos/1 -> x_dot/1, X_pos/1, Gain5/1  "x_dot"
  Add1/1 -> Gain4/1

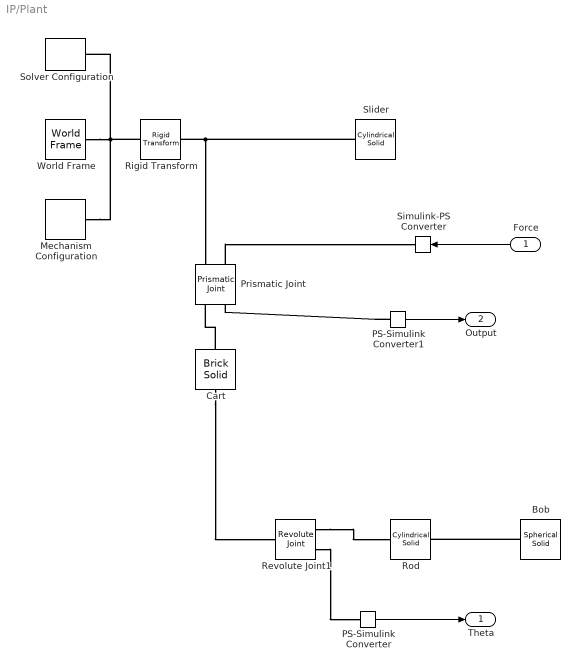
== system IP/Plant ==
  Force : Inport
  Bob : sm_lib/Body Elements/Spherical Solid  GraphicAmbientColor=[0.15 0.15 0.15 1.0]  BasedOnType=Density  CenterOfMass=[0 0 0]  CenterOfMassUnits=m  GraphicDiffuseColor=[1.0 0.4 0.4]  Density=1000  DensityUnits=kg/m^3  DoExposeReferenceFrame=on  GraphicEmissiveColor=[0.0 0.0 0.0 1.0]  ExportEntireGeometry=off  SerializedExposedGeometries=<ExposedGeometries/>  SerializedFrames=<Frames/>  MarkerShape=Sphere  MarkerSize=10  GraphicType=FromGeometry  InertiaType=PointMass  Mass=0.23  MassUnits=kg  MomentsOfInertia=[1 1 1]  MomentsOfInertiaUnits=kg*m^2  GraphicOpacity=1.0  ProductsOfInertia=[0 0 0]  ProductsOfInertiaUnits=kg*m^2  GraphicShininess=75  GraphicSpecularColor=[0.5 0.5 0.5 1.0]  SphereRadius=0.05  SphereRadiusUnits=m  GraphicVisPropType=SimpleVisualProperties
  Cart : sm_lib/Body Elements/Brick Solid  GraphicAmbientColor=[0.15 0.15 0.15 1.0]  BasedOnType=Density  BrickDimensions=[0.1 0.1 0.2]  BrickDimensionsUnits=m  CenterOfMass=[0 0 0]  CenterOfMassUnits=m  GraphicDiffuseColor=[1.0 0.6 0.2]  Density=1000  DensityUnits=kg/m^3  DoExposeReferenceFrame=on  GraphicEmissiveColor=[0.0 0.0 0.0 1.0]  ExportEntireGeometry=off  SerializedFrames=<Frames><Frame><Id>Frame2</Id><Value><Name>F2</Name><Origin><Source>GeometricFeature</Source><FeatureName>-x surface</FeatureName></Origin><PrimaryAxis><DefinedDirection>+Z</DefinedDirection><Source>ReferenceFrame</Source><SourceDirection>+Y</SourceDirection><FeatureName></FeatureName></PrimaryAxis><SecondaryAxis><DefinedDirection>+X</DefinedDirection><Source>ReferenceFrame</Source><SourceDirection>+X</SourceDirection><FeatureName></FeatureName></SecondaryAxis></Value></Frame></Frames>  MarkerShape=Sphere  MarkerSize=10  GraphicType=FromGeometry  InertiaType=PointMass  Mass=2.4  MassUnits=kg  MomentsOfInertia=[1 1 1]  MomentsOfInertiaUnits=kg*m^2  GraphicOpacity=0.5  ProductsOfInertia=[0 0 0]  ProductsOfInertiaUnits=kg*m^2  GraphicShininess=75  GraphicSpecularColor=[0.5 0.5 0.5 1.0]  GraphicVisPropType=SimpleVisualProperties
  Mechanism Configuration : sm_lib/Utilities/Mechanism Configuration  UniformGravity=Constant  GravityVector=[0 0 -9.80665]  GravityVectorUnits=m/s^2  LinearizationDelta=0.001  JointModeTransitionNonlinearIterations=2
  PS-Simulink Converter : nesl_utility/PS-Simulink Converter  PhysicalDomain=network_engine_domain  SubClassName=ps_output  LeftPortType=input  RightPortType=output  PseudoPeriodic=off  Frequencies=[]  VectorFormat=inherit  Unit=inherit  AffineConversion=off
  PS-Simulink Converter1 : nesl_utility/PS-Simulink Converter  PhysicalDomain=network_engine_domain  SubClassName=ps_output  LeftPortType=input  RightPortType=output  PseudoPeriodic=off  Frequencies=[]  VectorFormat=inherit  Unit=inherit  AffineConversion=off
  Prismatic Joint : sm_lib/Joints/Prismatic Joint  JointMode=Normal  SenseConstraintForce=off  SenseConstraintForceX=off  SenseConstraintForceY=off  SenseConstraintForceZ=off  SenseConstraintTorque=off  SenseConstraintTorqueX=off  SenseConstraintTorqueY=off  SenseConstraintTorqueZ=off  SenseTotalForce=off  SenseTotalForceX=off  SenseTotalForceY=off  SenseTotalForceZ=off  SenseTotalTorque=off  SenseTotalTorqueX=off  SenseTotalTorqueY=off  SenseTotalTorqueZ=off  CompositeWrenchDir=FollowerOnBase  CompositeWrenchFrame=BaseFrame  EquilibriumPosition=0  EquilibriumPositionUnits=m  SpringStiffness=0  SpringStiffnessUnits=N/m  DampingCoefficient=0.1  DampingCoefficientUnits=N/(m/s)  TorqueActuationMode=InputTorque  MotionActuationMode=ComputedMotion  SensePosition=off  SenseVelocity=on  SenseAcceleration=off  SenseTorqueForce=off  SenseLowerLimitTorqueForce=off  SenseUpperLimitTorqueForce=off  LowerLimitSpecify=off  LowerLimitBound=-1  LowerLimitBoundUnits=m  LowerLimitStiffness=1e6  LowerLimitStiffnessUnits=N/m  LowerLimitDamping=1e3  LowerLimitDampingUnits=N/(m/s)  LowerLimitTransitionRegionWidth=1e-4  LowerLimitTransitionRegionWidthUnits=m  UpperLimitSpecify=off  UpperLimitBound=1  UpperLimitBoundUnits=m  UpperLimitStiffness=1e6  UpperLimitStiffnessUnits=N/m  UpperLimitDamping=1e3  UpperLimitDampingUnits=N/(m/s)  UpperLimitTransitionRegionWidth=1e-4  UpperLimitTransitionRegionWidthUnits=m  PositionTargetSpecify=off  PositionTargetPriority=High  PositionTargetValue=0  PositionTargetValueUnits=m  VelocityTargetSpecify=off  VelocityTargetPriority=High  VelocityTargetValue=0  VelocityTargetValueUnits=m/s
  Revolute Joint1 : sm_lib/Joints/Revolute Joint  JointMode=Normal  SenseConstraintForce=off  SenseConstraintForceX=off  SenseConstraintForceY=off  SenseConstraintForceZ=off  SenseConstraintTorque=off  SenseConstraintTorqueX=off  SenseConstraintTorqueY=off  SenseConstraintTorqueZ=off  SenseTotalForce=off  SenseTotalForceX=off  SenseTotalForceY=off  SenseTotalForceZ=off  SenseTotalTorque=off  SenseTotalTorqueX=off  SenseTotalTorqueY=off  SenseTotalTorqueZ=off  CompositeWrenchDir=FollowerOnBase  CompositeWrenchFrame=BaseFrame  EquilibriumPosition=0  EquilibriumPositionUnits=deg  SpringStiffness=0  SpringStiffnessUnits=N*m/deg  DampingCoefficient=0  DampingCoefficientUnits=N*m/(deg/s)  TorqueActuationMode=NoTorque  MotionActuationMode=ComputedMotion  SensePosition=on  SenseVelocity=off  SenseAcceleration=off  SenseTorqueForce=off  SenseLowerLimitTorqueForce=off  SenseUpperLimitTorqueForce=off  LowerLimitSpecify=on  LowerLimitBound=-90  LowerLimitBoundUnits=deg  LowerLimitStiffness=1e4  LowerLimitStiffnessUnits=N*m/deg  LowerLimitDamping=10  LowerLimitDampingUnits=N*m/(deg/s)  LowerLimitTransitionRegionWidth=0.1  LowerLimitTransitionRegionWidthUnits=deg  UpperLimitSpecify=on  UpperLimitBound=90  UpperLimitBoundUnits=deg  UpperLimitStiffness=1e4  UpperLimitStiffnessUnits=N*m/deg  UpperLimitDamping=10  UpperLimitDampingUnits=N*m/(deg/s)  UpperLimitTransitionRegionWidth=0.1  UpperLimitTransitionRegionWidthUnits=deg  PositionTargetSpecify=off  PositionTargetPriority=High  PositionTargetValue=30  PositionTargetValueUnits=deg  VelocityTargetSpecify=off  VelocityTargetPriority=High  VelocityTargetValue=0  VelocityTargetValueUnits=deg/s
  Rigid Transform : sm_lib/Frames and Transforms/Rigid Transform  TranslationMethod=None  TranslationStandardOffset=0  TranslationStandardOffsetUnits=m  TranslationStandardAxis=+Z  TranslationCartesianOffset=[0 0 0]  TranslationCartesianOffsetUnits=m  TranslationROffset=0  TranslationROffsetUnits=m  TranslationZOffset=0  TranslationZOffsetUnits=m  TranslationThetaOffset=0  TranslationThetaOffsetUnits=deg  RotationMethod=StandardAxis  RotationAngleUnits=deg  RotationStandardAxis=+Y  RotationAngle=90  RotationArbitraryAxis=[0 0 1]  FollAlignAxisA=+X  BaseAlignAxisA=+Y  FollAlignAxisB=+Y  BaseAlignAxisB=+Z  RotationSequenceAxes=FollowerAxes  RotationSequence=XYX  RotationSequenceAngles=[0 0 0]  RotationSequenceAnglesUnits=deg  RotationMatrix=[1 0 0; 0 1 0; 0 0 1]  Quaternion=[1 0 0 0]
  Rod : sm_lib/Body Elements/Cylindrical Solid  GraphicAmbientColor=[0.15 0.15 0.15 1.0]  BasedOnType=Density  CenterOfMass=[0 0 0]  CenterOfMassUnits=m  GraphicDiffuseColor=[0.2 0.2 1.0]  CylinderLength=0.36  CylinderLengthUnits=m  CylinderRadius=0.01  CylinderRadiusUnits=m  Density=1000  DensityUnits=kg/m^3  DoExposeReferenceFrame=off  GraphicEmissiveColor=[0.0 0.0 0.0 1.0]  ExportEntireGeometry=off  SerializedFrames=<Frames><Frame><Id>Frame1</Id><Value><Name>F1</Name><Origin><Source>GeometricFeature</Source><FeatureName>bottom surface</FeatureName></Origin><PrimaryAxis><DefinedDirection>+Z</DefinedDirection><Source>ReferenceFrame</Source><SourceDirection>-Y</SourceDirection><FeatureName></FeatureName></PrimaryAxis><SecondaryAxis><DefinedDirection>+X</DefinedDirection><Source>ReferenceFrame</Source><SourceDirection>-Z</SourceDirection><FeatureName></FeatureName></SecondaryAxis></Value></Frame><Frame><Id>Frame2</Id><Value><Name>F2</Name><Origin><Source>GeometricFeature</Source><FeatureName>top curve</FeatureName></Origin><PrimaryAxis><DefinedDirection>+Z</DefinedDirection><Source>ReferenceFrame</Source><SourceDirection>-Y</SourceDirection><FeatureName></FeatureName></PrimaryAxis><SecondaryAxis><DefinedDirection>+X</DefinedDirection><Source>ReferenceFrame</Source><SourceDirection>+X</SourceDirection><FeatureName></FeatureName></SecondaryAxis></Value></Frame></Frames>  MarkerShape=Sphere  MarkerSize=10  GraphicType=FromGeometry  InertiaType=PointMass  Mass=0  MassUnits=kg  MomentsOfInertia=[1 1 1]  MomentsOfInertiaUnits=kg*m^2  GraphicOpacity=1.0  ProductsOfInertia=[0 0 0]  ProductsOfInertiaUnits=kg*m^2  GraphicShininess=75  GraphicSpecularColor=[0.5 0.5 0.5 1.0]  GraphicVisPropType=SimpleVisualProperties
  Simulink-PS Converter : nesl_utility/Simulink-PS Converter  PhysicalDomain=network_engine_domain  SubClassName=ps_input  LeftPortType=input  RightPortType=output  PseudoPeriodic=off  Frequencies=[]  NoiseDistribution=none  NoiseParameters=[]  Unit=1  AffineConversion=off  FilteringAndDerivatives=provide  SimscapeFilterOrder=1  InputFilterTimeConstant=0.001  UdotUserProvided=0
  Slider : sm_lib/Body Elements/Cylindrical Solid  GraphicAmbientColor=[0.15 0.15 0.15 1.0]  BasedOnType=Density  CenterOfMass=[0 0 0]  CenterOfMassUnits=m  GraphicDiffuseColor=[0.5 0.5 0.5]  CylinderLength=1  CylinderLengthUnits=m  CylinderRadius=0.01  CylinderRadiusUnits=m  Density=1000  DensityUnits=kg/m^3  DoExposeReferenceFrame=on  GraphicEmissiveColor=[0.0 0.0 0.0 1.0]  ExportEntireGeometry=off  SerializedFrames=<Frames/>  MarkerShape=Sphere  MarkerSize=10  GraphicType=FromGeometry  InertiaType=PointMass  Mass=5  MassUnits=kg  MomentsOfInertia=[1 1 1]  MomentsOfInertiaUnits=kg*m^2  GraphicOpacity=1.0  ProductsOfInertia=[0 0 0]  ProductsOfInertiaUnits=kg*m^2  GraphicShininess=75  GraphicSpecularColor=[0.5 0.5 0.5 1.0]  GraphicVisPropType=SimpleVisualProperties
  Solver Configuration : nesl_utility/Solver Configuration  PhysicalDomain=network_engine_domain  SubClassName=solver  LeftPortType=input  RightPortType=generic  Tones=[]  Harmonics=[]  SimulateNoise=off  Profile=off  UseLocalSampling=off  EnableSwitchedLinearOptims=on  FrequencyDomain=off  UseCCode=off  RelTol=0.001  AbsTol=1e-06  MinStep=1e-09  ToWorkspace=off  RevertToSquareIcSolve=off  NumHomotopyIterations=100  PhasorMode=off  PhasorModeNumHarmonics=1  ConsistencySolver=NEWTON_XTOL_AFTER_FTOL  IndexReductionMethod=DerivativeReplacement  DoDC=off  ResidualTolerance=1e-09  ConsistencyTolSource=GLOBAL  ConsistencyAbsTol=0.001  ConsistencyRelTol=0.001  ConsistencyTolFactor=0.001  UseLocalSolver=off  LocalSolverChoice=NE_BACKWARD_EULER_ADVANCER  ResolveIndetEquations=on  FunctionEvalNumThread=1  LocalSolverSampleTime=0.001  DoFixedCost=off  MaxNonlinIter=3  MaxModeIter=2  ComputeImpulses=off  ImpulseIterations=2  LinearAlgebra=Sparse  LinearAlgebraNumThread=0  EquationFormulation=NE_TIME_EF  DelaysMemoryBudget=1024  AutomaticFiltering=on  FilteringTimeConstant=0.001  PartitionStorageMethod=AS_NEEDED  PartitionMemoryBudget=1024  PartitionMethod=FAST
  World Frame : sm_lib/Frames and Transforms/World Frame
  Theta : Outport
  Output : Outport  Port=2
  wires:
  Force/1 -> Simulink-PS Converter/1
  PS-Simulink Converter/1 -> Theta/1
  PS-Simulink Converter1/1 -> Output/1
  connections:
  Slider/RConn1 -- Rigid Transform/RConn1 -- Prismatic Joint/LConn1
  Bob/RConn1 -- Rod/RConn1
  Revolute Joint1/RConn1 -- Rod/LConn1
  World Frame/RConn1 -- Solver Configuration/RConn1 -- Rigid Transform/LConn1 -- Mechanism Configuration/RConn1
  Cart/LConn1 -- Revolute Joint1/LConn1
  Prismatic Joint/LConn2 -- Simulink-PS Converter/RConn1
  Cart/RConn1 -- Prismatic Joint/RConn1
  Revolute Joint1/RConn2 -- PS-Simulink Converter/LConn1
  PS-Simulink Converter1/LConn1 -- Prismatic Joint/RConn2
